simulink model "Appl_VentAdj_CtrlModel"  (R2018b)
settings: configuration reference "CodeConfig_10_ms" (kept outside this file)
undefined symbols (not defined in the file): D_VENT_LVL_1_PRECENT, D_VENT_LVL_2_PRECENT, D_VENT_LVL_3_PRECENT, FALSE, TRUE
libraries: DareLib x72, simulink x1
(part 2 of 4)

== system Appl_VentAdj_CtrlModel/LogicCtrl/LocalAdjustCtrl/LimitDeal/LevelLimitFunction2 ==
  OriginalLevel : Inport
  Error : Inport  Port=2
  OppositeCmd : Inport  Port=3
  CarType : Inport  Port=4
  Vent_CanMessageLostFlag : Inport  Port=5
  Vent_RecoverDefaultFlag : Inport  Port=6
  f : TriggerPort  TriggerType=function-call  VariantControl=(inherit)
      settings: CopyFcn=Stateflow.SLINSF.SimulinkMan.removeBlockPreDeleteFcn  PreDeleteFcn=Stateflow.SLINSF.SimulinkMan.unsafePredeleteFcn
  LevelLimit : Stateflow chart  TreatAsAtomicUnit=on
  Level : Outport
  StopReason : Outport  Port=2
  wires:
  OriginalLevel/1 -> LevelLimit/1(OriginalLevel)
  Error/1 -> LevelLimit/2(Error)
  CarType/1 -> LevelLimit/3(CarType)
  OppositeCmd/1 -> LevelLimit/4(OppositeCmd)
  Vent_CanMessageLostFlag/1 -> LevelLimit/5(Vent_CanMessageLostFlag)
  Vent_RecoverDefaultFlag/1 -> LevelLimit/6(Vent_RecoverDefaultFlag)
  LevelLimit/1(Level) -> Level/1
  LevelLimit/2(StopReason) -> StopReason/1

== system Appl_VentAdj_CtrlModel/LogicCtrl/LocalAdjustCtrl/LimitDeal/MixConflic ==
  MixFlg : Inport  OutDataTypeStr=uint8
  Valid : Inport  Port=2  OutDataTypeStr=uint8
  f : TriggerPort  TriggerType=function-call  VariantControl=(inherit)
      settings: CopyFcn=Stateflow.SLINSF.SimulinkMan.removeBlockPreDeleteFcn  PreDeleteFcn=Stateflow.SLINSF.SimulinkMan.unsafePredeleteFcn
  Constant : Constant  Value=FALSE
  Switch : Switch  Criteria=u2 ~= 0  OutDataTypeStr=uint8
  OutValid : Outport
  wires:
  MixFlg/1 -> Switch/2
  Constant/1 -> Switch/1
  Valid/1 -> Switch/3
  Switch/1 -> OutValid/1

== system Appl_VentAdj_CtrlModel/LogicCtrl/LocalAdjustCtrl/LimitDeal/StopFunction ==
  ComStop : Inport
  Timeout : Inport  Port=2
  f : TriggerPort  TriggerType=function-call  VariantControl=(inherit)
      settings: CopyFcn=Stateflow.SLINSF.SimulinkMan.removeBlockPreDeleteFcn  PreDeleteFcn=Stateflow.SLINSF.SimulinkMan.unsafePredeleteFcn
  StopFunction : Stateflow chart  TreatAsAtomicUnit=on
  StopReason : Outport
  wires:
  Timeout/1 -> StopFunction/1(Timeout)
  ComStop/1 -> StopFunction/2(ComStop)
  StopFunction/1(StopReason) -> StopReason/1

== system Appl_VentAdj_CtrlModel/LogicCtrl/LocalAdjustCtrl/LimitDeal/StopFunction1 ==
  ComStop : Inport
  Timeout : Inport  Port=2
  f : TriggerPort  TriggerType=function-call  VariantControl=(inherit)
      settings: CopyFcn=Stateflow.SLINSF.SimulinkMan.removeBlockPreDeleteFcn  PreDeleteFcn=Stateflow.SLINSF.SimulinkMan.unsafePredeleteFcn
  StopFunction : Stateflow chart  TreatAsAtomicUnit=on
  StopReason : Outport
  wires:
  Timeout/1 -> StopFunction/1(Timeout)
  ComStop/1 -> StopFunction/2(ComStop)
  StopFunction/1(StopReason) -> StopReason/1

== system Appl_VentAdj_CtrlModel/LogicCtrl/LocalAdjustCtrl/LimitDeal/StopFunction2 ==
  ComStop : Inport
  Timeout : Inport  Port=2
  f : TriggerPort  TriggerType=function-call  VariantControl=(inherit)
      settings: CopyFcn=Stateflow.SLINSF.SimulinkMan.removeBlockPreDeleteFcn  PreDeleteFcn=Stateflow.SLINSF.SimulinkMan.unsafePredeleteFcn
  StopFunction : Stateflow chart  TreatAsAtomicUnit=on
  StopReason : Outport
  wires:
  Timeout/1 -> StopFunction/1(Timeout)
  ComStop/1 -> StopFunction/2(ComStop)
  StopFunction/1(StopReason) -> StopReason/1

== system Appl_VentAdj_CtrlModel/LogicCtrl/LocalAdjustCtrl/LimitDeal/TimeoutFunction ==
  TimeoutPrm : Inport
  MaxTime : Inport  Port=2  OutDataTypeStr=uint32
  InLevel : Inport  Port=3
  f : TriggerPort  TriggerType=function-call  VariantControl=(inherit)
      settings: CopyFcn=Stateflow.SLINSF.SimulinkMan.removeBlockPreDeleteFcn  PreDeleteFcn=Stateflow.SLINSF.SimulinkMan.unsafePredeleteFcn
  Timeout : Stateflow chart  TreatAsAtomicUnit=on
  Level : Outport
  TimeoutFlag : Outport  Port=2
  wires:
  TimeoutPrm/1 -> Timeout/1(TimeoutPrm)
  InLevel/1 -> Timeout/2(InLevel)
  Timeout/2(Level) -> Level/1
  Timeout/1(TimeoutFlag) -> TimeoutFlag/1
  MaxTime/1 -> Timeout/3(MaxTime)

== system Appl_VentAdj_CtrlModel/LogicCtrl/LocalAdjustCtrl/LimitDeal/TimeoutFunction1 ==
  TimeoutPrm : Inport
  MaxTime : Inport  Port=2  OutDataTypeStr=uint32
  InLevel : Inport  Port=3
  f : TriggerPort  TriggerType=function-call  VariantControl=(inherit)
      settings: CopyFcn=Stateflow.SLINSF.SimulinkMan.removeBlockPreDeleteFcn  PreDeleteFcn=Stateflow.SLINSF.SimulinkMan.unsafePredeleteFcn
  Timeout : Stateflow chart  TreatAsAtomicUnit=on
  Level : Outport
  TimeoutFlag : Outport  Port=2
  wires:
  TimeoutPrm/1 -> Timeout/1(TimeoutPrm)
  InLevel/1 -> Timeout/2(InLevel)
  Timeout/2(Level) -> Level/1
  Timeout/1(TimeoutFlag) -> TimeoutFlag/1
  MaxTime/1 -> Timeout/3(MaxTime)

== system Appl_VentAdj_CtrlModel/LogicCtrl/LocalAdjustCtrl/LimitDeal/TimeoutFunction2 ==
  TimeoutPrm : Inport
  MaxTime : Inport  Port=2  OutDataTypeStr=uint32
  InLevel : Inport  Port=3
  f : TriggerPort  TriggerType=function-call  VariantControl=(inherit)
      settings: CopyFcn=Stateflow.SLINSF.SimulinkMan.removeBlockPreDeleteFcn  PreDeleteFcn=Stateflow.SLINSF.SimulinkMan.unsafePredeleteFcn
  Timeout : Stateflow chart  TreatAsAtomicUnit=on
  Level : Outport
  TimeoutFlag : Outport  Port=2
  wires:
  TimeoutPrm/1 -> Timeout/1(TimeoutPrm)
  InLevel/1 -> Timeout/2(InLevel)
  Timeout/2(Level) -> Level/1
  Timeout/1(TimeoutFlag) -> TimeoutFlag/1
  MaxTime/1 -> Timeout/3(MaxTime)

== system Appl_VentAdj_CtrlModel/LogicCtrl/LocalAdjustCtrl/OutputDeal/DutyFunction ==
  AimLevel : Inport
  f : TriggerPort  TriggerType=function-call  VariantControl=(inherit)
      settings: CopyFcn=Stateflow.SLINSF.SimulinkMan.removeBlockPreDeleteFcn  PreDeleteFcn=Stateflow.SLINSF.SimulinkMan.unsafePredeleteFcn
  Duty : Stateflow chart  TreatAsAtomicUnit=on
  AimDuty : Outport
  wires:
  AimLevel/1 -> Duty/1(AimLevel)
  Duty/1(AimDuty) -> AimDuty/1

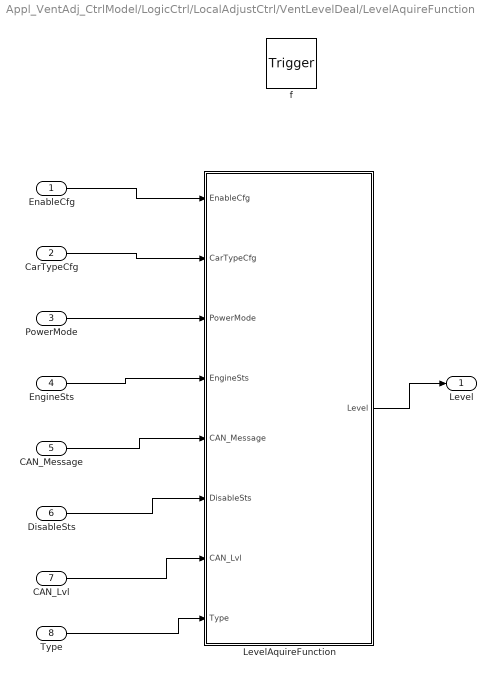
== system Appl_VentAdj_CtrlModel/LogicCtrl/LocalAdjustCtrl/VentLevelDeal/LevelAquireFunction ==
  EnableCfg : Inport
  CarTypeCfg : Inport  Port=2
  PowerMode : Inport  Port=3
  EngineSts : Inport  Port=4
  CAN_Message : Inport  Port=5
  DisableSts : Inport  Port=6
  CAN_Lvl : Inport  Port=7
  Type : Inport  Port=8  OutDataTypeStr=uint8
  f : TriggerPort  TriggerType=function-call  VariantControl=(inherit)
      settings: CopyFcn=Stateflow.SLINSF.SimulinkMan.removeBlockPreDeleteFcn  PreDeleteFcn=Stateflow.SLINSF.SimulinkMan.unsafePredeleteFcn
  LevelAquireFunction : Stateflow chart  TreatAsAtomicUnit=on
  "Level " : Outport
  wires:
  EnableCfg/1 -> LevelAquireFunction/1(EnableCfg)
  DisableSts/1 -> LevelAquireFunction/6(DisableSts)
  CarTypeCfg/1 -> LevelAquireFunction/2(CarTypeCfg)
  CAN_Message/1 -> LevelAquireFunction/5(CAN_Message)
  EngineSts/1 -> LevelAquireFunction/4(EngineSts)
  PowerMode/1 -> LevelAquireFunction/3(PowerMode)
  LevelAquireFunction/1(Level) -> "Level "/1
  CAN_Lvl/1 -> LevelAquireFunction/7(CAN_Lvl)
  Type/1 -> LevelAquireFunction/8(Type)

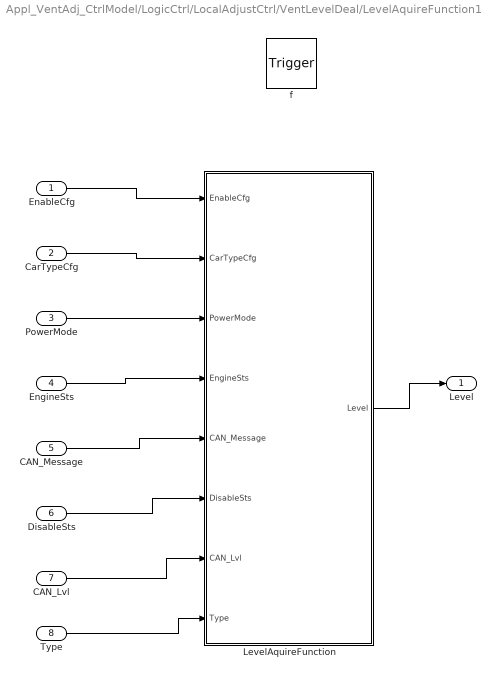
== system Appl_VentAdj_CtrlModel/LogicCtrl/LocalAdjustCtrl/VentLevelDeal/LevelAquireFunction1 ==
  EnableCfg : Inport
  CarTypeCfg : Inport  Port=2
  PowerMode : Inport  Port=3
  EngineSts : Inport  Port=4
  CAN_Message : Inport  Port=5
  DisableSts : Inport  Port=6
  CAN_Lvl : Inport  Port=7
  Type : Inport  Port=8  OutDataTypeStr=uint8
  f : TriggerPort  TriggerType=function-call  VariantControl=(inherit)
      settings: CopyFcn=Stateflow.SLINSF.SimulinkMan.removeBlockPreDeleteFcn  PreDeleteFcn=Stateflow.SLINSF.SimulinkMan.unsafePredeleteFcn
  LevelAquireFunction : Stateflow chart  TreatAsAtomicUnit=on
  "Level " : Outport
  wires:
  EnableCfg/1 -> LevelAquireFunction/1(EnableCfg)
  DisableSts/1 -> LevelAquireFunction/6(DisableSts)
  CarTypeCfg/1 -> LevelAquireFunction/2(CarTypeCfg)
  CAN_Message/1 -> LevelAquireFunction/5(CAN_Message)
  EngineSts/1 -> LevelAquireFunction/4(EngineSts)
  PowerMode/1 -> LevelAquireFunction/3(PowerMode)
  LevelAquireFunction/1(Level) -> "Level "/1
  CAN_Lvl/1 -> LevelAquireFunction/7(CAN_Lvl)
  Type/1 -> LevelAquireFunction/8(Type)

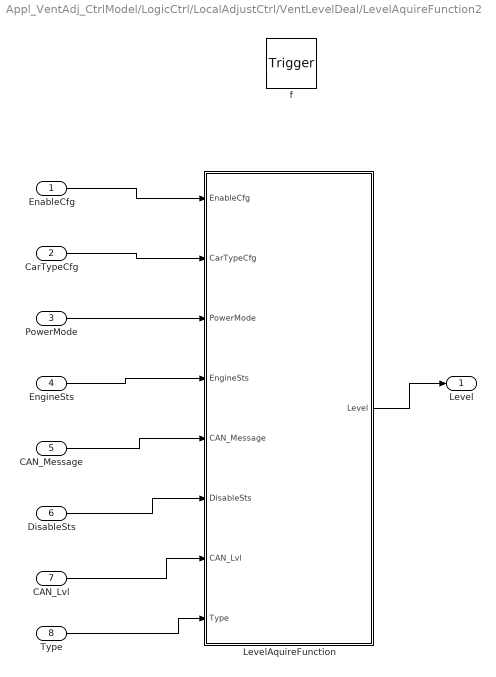
== system Appl_VentAdj_CtrlModel/LogicCtrl/LocalAdjustCtrl/VentLevelDeal/LevelAquireFunction2 ==
  EnableCfg : Inport
  CarTypeCfg : Inport  Port=2
  PowerMode : Inport  Port=3
  EngineSts : Inport  Port=4
  CAN_Message : Inport  Port=5
  DisableSts : Inport  Port=6
  CAN_Lvl : Inport  Port=7
  Type : Inport  Port=8  OutDataTypeStr=uint8
  f : TriggerPort  TriggerType=function-call  VariantControl=(inherit)
      settings: CopyFcn=Stateflow.SLINSF.SimulinkMan.removeBlockPreDeleteFcn  PreDeleteFcn=Stateflow.SLINSF.SimulinkMan.unsafePredeleteFcn
  LevelAquireFunction : Stateflow chart  TreatAsAtomicUnit=on
  "Level " : Outport
  wires:
  EnableCfg/1 -> LevelAquireFunction/1(EnableCfg)
  DisableSts/1 -> LevelAquireFunction/6(DisableSts)
  CarTypeCfg/1 -> LevelAquireFunction/2(CarTypeCfg)
  CAN_Message/1 -> LevelAquireFunction/5(CAN_Message)
  EngineSts/1 -> LevelAquireFunction/4(EngineSts)
  PowerMode/1 -> LevelAquireFunction/3(PowerMode)
  LevelAquireFunction/1(Level) -> "Level "/1
  CAN_Lvl/1 -> LevelAquireFunction/7(CAN_Lvl)
  Type/1 -> LevelAquireFunction/8(Type)

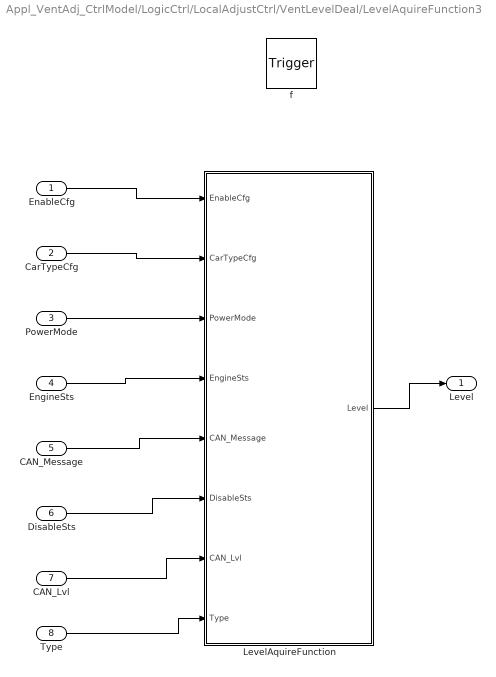
== system Appl_VentAdj_CtrlModel/LogicCtrl/LocalAdjustCtrl/VentLevelDeal/LevelAquireFunction3 ==
  EnableCfg : Inport
  CarTypeCfg : Inport  Port=2
  PowerMode : Inport  Port=3
  EngineSts : Inport  Port=4
  CAN_Message : Inport  Port=5
  DisableSts : Inport  Port=6
  CAN_Lvl : Inport  Port=7
  Type : Inport  Port=8  OutDataTypeStr=uint8
  f : TriggerPort  TriggerType=function-call  VariantControl=(inherit)
      settings: CopyFcn=Stateflow.SLINSF.SimulinkMan.removeBlockPreDeleteFcn  PreDeleteFcn=Stateflow.SLINSF.SimulinkMan.unsafePredeleteFcn
  LevelAquireFunction : Stateflow chart  TreatAsAtomicUnit=on
  "Level " : Outport
  wires:
  EnableCfg/1 -> LevelAquireFunction/1(EnableCfg)
  DisableSts/1 -> LevelAquireFunction/6(DisableSts)
  CarTypeCfg/1 -> LevelAquireFunction/2(CarTypeCfg)
  CAN_Message/1 -> LevelAquireFunction/5(CAN_Message)
  EngineSts/1 -> LevelAquireFunction/4(EngineSts)
  PowerMode/1 -> LevelAquireFunction/3(PowerMode)
  LevelAquireFunction/1(Level) -> "Level "/1
  CAN_Lvl/1 -> LevelAquireFunction/7(CAN_Lvl)
  Type/1 -> LevelAquireFunction/8(Type)

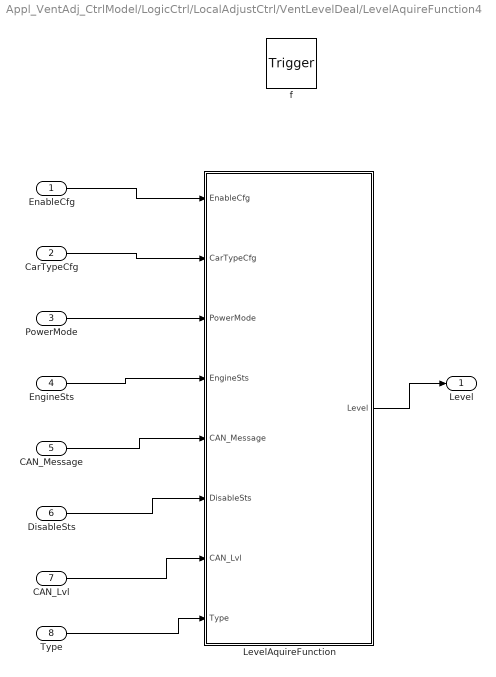
== system Appl_VentAdj_CtrlModel/LogicCtrl/LocalAdjustCtrl/VentLevelDeal/LevelAquireFunction4 ==
  EnableCfg : Inport
  CarTypeCfg : Inport  Port=2
  PowerMode : Inport  Port=3
  EngineSts : Inport  Port=4
  CAN_Message : Inport  Port=5
  DisableSts : Inport  Port=6
  CAN_Lvl : Inport  Port=7
  Type : Inport  Port=8  OutDataTypeStr=uint8
  f : TriggerPort  TriggerType=function-call  VariantControl=(inherit)
      settings: CopyFcn=Stateflow.SLINSF.SimulinkMan.removeBlockPreDeleteFcn  PreDeleteFcn=Stateflow.SLINSF.SimulinkMan.unsafePredeleteFcn
  LevelAquireFunction : Stateflow chart  TreatAsAtomicUnit=on
  "Level " : Outport
  wires:
  EnableCfg/1 -> LevelAquireFunction/1(EnableCfg)
  DisableSts/1 -> LevelAquireFunction/6(DisableSts)
  CarTypeCfg/1 -> LevelAquireFunction/2(CarTypeCfg)
  CAN_Message/1 -> LevelAquireFunction/5(CAN_Message)
  EngineSts/1 -> LevelAquireFunction/4(EngineSts)
  PowerMode/1 -> LevelAquireFunction/3(PowerMode)
  LevelAquireFunction/1(Level) -> "Level "/1
  CAN_Lvl/1 -> LevelAquireFunction/7(CAN_Lvl)
  Type/1 -> LevelAquireFunction/8(Type)

== system Appl_VentAdj_CtrlModel/LogicCtrl/LocalAdjustCtrl/VentLevelDeal/LevelAquireFunction5 ==
  EnableCfg : Inport
  CarTypeCfg : Inport  Port=2
  PowerMode : Inport  Port=3
  EngineSts : Inport  Port=4
  CAN_Message : Inport  Port=5
  DisableSts : Inport  Port=6
  CAN_Lvl : Inport  Port=7
  Type : Inport  Port=8  OutDataTypeStr=uint8
  f : TriggerPort  TriggerType=function-call  VariantControl=(inherit)
      settings: CopyFcn=Stateflow.SLINSF.SimulinkMan.removeBlockPreDeleteFcn  PreDeleteFcn=Stateflow.SLINSF.SimulinkMan.unsafePredeleteFcn
  LevelAquireFunction : Stateflow chart  TreatAsAtomicUnit=on
  "Level " : Outport
  wires:
  EnableCfg/1 -> LevelAquireFunction/1(EnableCfg)
  DisableSts/1 -> LevelAquireFunction/6(DisableSts)
  CarTypeCfg/1 -> LevelAquireFunction/2(CarTypeCfg)
  CAN_Message/1 -> LevelAquireFunction/5(CAN_Message)
  EngineSts/1 -> LevelAquireFunction/4(EngineSts)
  PowerMode/1 -> LevelAquireFunction/3(PowerMode)
  LevelAquireFunction/1(Level) -> "Level "/1
  CAN_Lvl/1 -> LevelAquireFunction/7(CAN_Lvl)
  Type/1 -> LevelAquireFunction/8(Type)

== system Appl_VentAdj_CtrlModel/LogicCtrl/LocalAdjustCtrl/VentLevelDeal/VentRunTypeFunction ==
  InLevel : Inport
  PreLevel : Inport  Port=2
  InType : Inport  Port=3
  f : TriggerPort  TriggerType=function-call  VariantControl=(inherit)
      settings: CopyFcn=Stateflow.SLINSF.SimulinkMan.removeBlockPreDeleteFcn  PreDeleteFcn=Stateflow.SLINSF.SimulinkMan.unsafePredeleteFcn
  VentRunType : Stateflow chart  TreatAsAtomicUnit=on
  RunType : Outport
  OutLevel : Outport  Port=2
  wires:
  InLevel/1 -> VentRunType/1(InLevel)
  PreLevel/1 -> VentRunType/2(PreLevel)
  InType/1 -> VentRunType/3(InType)
  VentRunType/1(RunType) -> RunType/1
  VentRunType/2(OutLevel) -> OutLevel/1

== system Appl_VentAdj_CtrlModel/UpDataInputInfo/InputSignalProcess/CommonPreconditionDeal ==
  EngineRunningFlag : Inport
  VehicleRunFlag : Inport  Port=2
  VentAdj_VoltMode : Inport  Port=3
  Deal : Stateflow chart  TreatAsAtomicUnit=on
  "ComPCSatisfiedFlag " : Outport
  wires:
  EngineRunningFlag/1 -> Deal/1(EngineRunningFlag)
  VehicleRunFlag/1 -> Deal/2(VehicleRunFlag)
  Deal/1(ComPCSatisfiedFlag) -> "ComPCSatisfiedFlag "/1
  VentAdj_VoltMode/1 -> Deal/3(VentAdj_VoltMode)

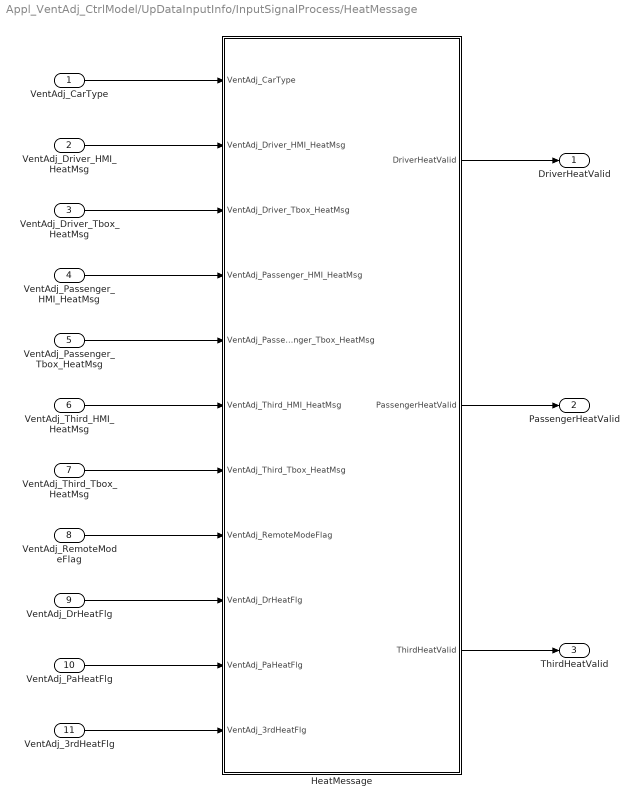
== system Appl_VentAdj_CtrlModel/UpDataInputInfo/InputSignalProcess/HeatMessage ==
  VentAdj_CarType : Inport
  VentAdj_Driver_HMI_HeatMsg : Inport  Port=2
  VentAdj_Driver_Tbox_HeatMsg : Inport  Port=3
  VentAdj_Passenger_HMI_HeatMsg : Inport  Port=4
  VentAdj_Passenger_Tbox_HeatMsg : Inport  Port=5
  VentAdj_Third_HMI_HeatMsg : Inport  Port=6
  VentAdj_Third_Tbox_HeatMsg : Inport  Port=7
  VentAdj_RemoteModeFlag : Inport  Port=8
  VentAdj_DrHeatFlg : Inport  Port=9
  VentAdj_PaHeatFlg : Inport  Port=10
  VentAdj_3rdHeatFlg : Inport  Port=11
  HeatMessage : Stateflow chart  TreatAsAtomicUnit=on
  DriverHeatValid : Outport
  PassengerHeatValid : Outport  Port=2
  ThirdHeatValid : Outport  Port=3
  wires:
  VentAdj_Driver_HMI_HeatMsg/1 -> HeatMessage/2(VentAdj_Driver_HMI_HeatMsg)
  VentAdj_CarType/1 -> HeatMessage/1(VentAdj_CarType)
  VentAdj_Driver_Tbox_HeatMsg/1 -> HeatMessage/3(VentAdj_Driver_Tbox_HeatMsg)
  VentAdj_Passenger_HMI_HeatMsg/1 -> HeatMessage/4(VentAdj_Passenger_HMI_HeatMsg)
  VentAdj_Passenger_Tbox_HeatMsg/1 -> HeatMessage/5(VentAdj_Passenger_Tbox_HeatMsg)
  VentAdj_RemoteModeFlag/1 -> HeatMessage/8(VentAdj_RemoteModeFlag)
  VentAdj_Third_HMI_HeatMsg/1 -> HeatMessage/6(VentAdj_Third_HMI_HeatMsg)
  VentAdj_Third_Tbox_HeatMsg/1 -> HeatMessage/7(VentAdj_Third_Tbox_HeatMsg)
  HeatMessage/1(DriverHeatValid) -> DriverHeatValid/1
  HeatMessage/2(PassengerHeatValid) -> PassengerHeatValid/1
  HeatMessage/3(ThirdHeatValid) -> ThirdHeatValid/1
  VentAdj_DrHeatFlg/1 -> HeatMessage/9(VentAdj_DrHeatFlg)
  VentAdj_PaHeatFlg/1 -> HeatMessage/10(VentAdj_PaHeatFlg)
  VentAdj_3rdHeatFlg/1 -> HeatMessage/11(VentAdj_3rdHeatFlg)

== system Appl_VentAdj_CtrlModel/UpDataInputInfo/InputSignalProcess/MaxTime ==
  VentAdj_CarType : Inport
  Constant : Constant  Value=60  OutDataTypeStr=uint32
  Constant1 : Constant  Value=1000  OutDataTypeStr=uint32
  Constant5 : Constant  Value=[0 0]  OutDataTypeStr=uint32
  Product : Product  Inputs=3  OutDataTypeStr=uint32
  Selector5 : Selector  IndexMode=Zero-based  InputPortWidth=2  IndexOptions=Index vector (port)  Indices=[1 3]  OutputSizes=1
  TimeChangeToCycle5 : DareLib/Dare/TimeChangeToCycle  Description=时间转成执行周期  Commented=on  Sec=60  Msec=1000  Cycle=CAL_HeatAdjCycle_10ms
      settings: AttributesFormatString=%<Description>  SourceProductName=Dare Library
  VentRunMaxTime : Outport
  wires:
  VentAdj_CarType/1 -> Selector5/2
  Constant5/1 -> Selector5/1
  Selector5/1 -> Product/2
  Constant/1 -> Product/1
  Constant1/1 -> Product/3
  Product/1 -> VentRunMaxTime/1

== system Appl_VentAdj_CtrlModel/UpDataInputInfo/InputSignalProcess/Subsystem ==
  VentAdj_DriverEnableConfig : Inport
  VentAdj_PassengerEnableConfig : Inport  Port=2
  VentAdj_ThirdEnableConfig : Inport  Port=3
  VentAdj_DrVentFlg : Inport  Port=4
  VentAdj_PaVentFlg : Inport  Port=5
  Bus Creator : BusCreator  Inputs=3
  Logical Operator : Logic  AllPortsSameDT=off  OutDataTypeStr=boolean
  Logical Operator1 : Logic  AllPortsSameDT=off  OutDataTypeStr=boolean
  VentEnable : Outport
  wires:
  Bus Creator/1 -> VentEnable/1
  VentAdj_DriverEnableConfig/1 -> Logical Operator1/1
  Logical Operator1/1 -> Bus Creator/1  "DrvVentFlg"
  VentAdj_PaVentFlg/1 -> Logical Operator/2
  VentAdj_PassengerEnableConfig/1 -> Logical Operator/1
  Logical Operator/1 -> Bus Creator/2  "PaVentFlg"
  VentAdj_ThirdEnableConfig/1 -> Bus Creator/3  "ThirdVentFlg"
  VentAdj_DrVentFlg/1 -> Logical Operator1/2

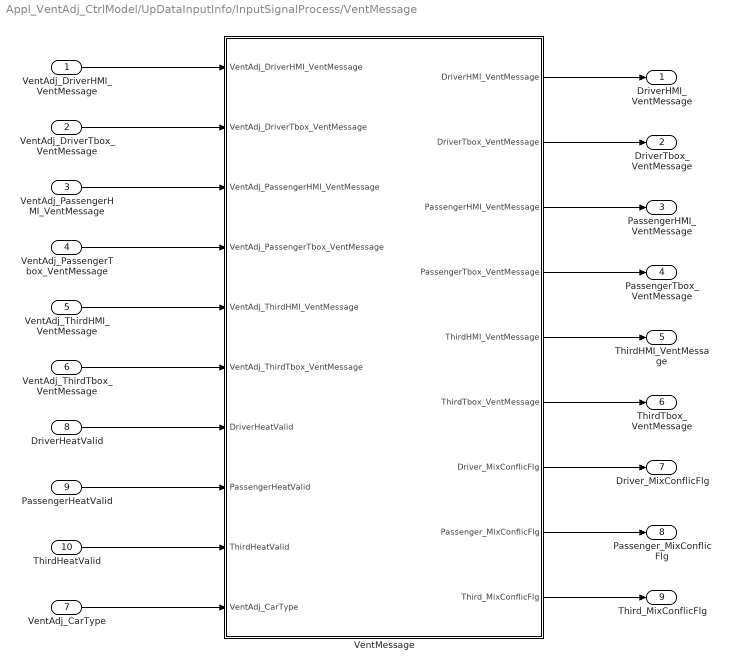
== system Appl_VentAdj_CtrlModel/UpDataInputInfo/InputSignalProcess/VentMessage ==
  VentAdj_DriverHMI_VentMessage : Inport
  VentAdj_DriverTbox_VentMessage : Inport  Port=2
  VentAdj_PassengerHMI_VentMessage : Inport  Port=3
  VentAdj_PassengerTbox_VentMessage : Inport  Port=4
  VentAdj_ThirdHMI_VentMessage : Inport  Port=5
  VentAdj_ThirdTbox_VentMessage : Inport  Port=6
  VentAdj_CarType : Inport  Port=7
  DriverHeatValid : Inport  Port=8
  PassengerHeatValid : Inport  Port=9
  ThirdHeatValid : Inport  Port=10
  VentMessage : Stateflow chart  TreatAsAtomicUnit=on
  DriverHMI_VentMessage : Outport
  DriverTbox_VentMessage : Outport  Port=2
  PassengerHMI_VentMessage : Outport  Port=3
  PassengerTbox_VentMessage : Outport  Port=4
  ThirdHMI_VentMessage : Outport  Port=5
  ThirdTbox_VentMessage : Outport  Port=6
  Driver_MixConflicFlg : Outport  Port=7
  Passenger_MixConflicFlg : Outport  Port=8
  Third_MixConflicFlg : Outport  Port=9
  wires:
  VentMessage/3(PassengerHMI_VentMessage) -> PassengerHMI_VentMessage/1
  VentMessage/2(DriverTbox_VentMessage) -> DriverTbox_VentMessage/1
  VentMessage/1(DriverHMI_VentMessage) -> DriverHMI_VentMessage/1
  DriverHeatValid/1 -> VentMessage/7(DriverHeatValid)
  VentAdj_ThirdTbox_VentMessage/1 -> VentMessage/6(VentAdj_ThirdTbox_VentMessage)
  PassengerHeatValid/1 -> VentMessage/8(PassengerHeatValid)
  VentAdj_ThirdHMI_VentMessage/1 -> VentMessage/5(VentAdj_ThirdHMI_VentMessage)
  VentAdj_PassengerTbox_VentMessage/1 -> VentMessage/4(VentAdj_PassengerTbox_VentMessage)
  VentAdj_PassengerHMI_VentMessage/1 -> VentMessage/3(VentAdj_PassengerHMI_VentMessage)
  VentAdj_DriverHMI_VentMessage/1 -> VentMessage/1(VentAdj_DriverHMI_VentMessage)
  VentAdj_DriverTbox_VentMessage/1 -> VentMessage/2(VentAdj_DriverTbox_VentMessage)
  ThirdHeatValid/1 -> VentMessage/9(ThirdHeatValid)
  VentMessage/6(ThirdTbox_VentMessage) -> ThirdTbox_VentMessage/1
  VentMessage/5(ThirdHMI_VentMessage) -> ThirdHMI_VentMessage/1
  VentMessage/4(PassengerTbox_VentMessage) -> PassengerTbox_VentMessage/1
  VentAdj_CarType/1 -> VentMessage/10(VentAdj_CarType)
  VentMessage/7(Driver_MixConflicFlg) -> Driver_MixConflicFlg/1
  VentMessage/8(Passenger_MixConflicFlg) -> Passenger_MixConflicFlg/1
  VentMessage/9(Third_MixConflicFlg) -> Third_MixConflicFlg/1

== system Appl_VentAdj_CtrlModel/LogicCtrl/LocalAdjustCtrl/LimitDeal/TimeoutFunction/Timeout/D_HAL_GET_CUR_MS_TS ==
  f : TriggerPort  TriggerType=function-call  VariantControl=(inherit)
      settings: CopyFcn=Stateflow.SLINSF.SimulinkMan.removeBlockPreDeleteFcn  PreDeleteFcn=Stateflow.SLINSF.SimulinkMan.unsafePredeleteFcn
  DrAdj_LenAdjSize : DareLib/Dare/getAPI_type  g_funcname=D_HAL_GET_CUR_MS_TS  g_param=""  g_type=uint32  g_size=-1
      settings: SourceProductName=Dare Library
  Ts : Outport
  wires:
  DrAdj_LenAdjSize/1 -> Ts/1  "D_HAL_GET_CUR_MS_TS"

== system Appl_VentAdj_CtrlModel/LogicCtrl/LocalAdjustCtrl/LimitDeal/TimeoutFunction/Timeout/TimeDiffTs ==
  lastTs : Inport
  Ts : Inport  Port=2
  f : TriggerPort  TriggerType=function-call  VariantControl=(inherit)
      settings: CopyFcn=Stateflow.SLINSF.SimulinkMan.removeBlockPreDeleteFcn  PreDeleteFcn=Stateflow.SLINSF.SimulinkMan.unsafePredeleteFcn
  Chart : Stateflow chart  TreatAsAtomicUnit=on
  OutTs : Outport
  wires:
  lastTs/1 -> Chart/1(lastTs)
  Ts/1 -> Chart/2(Ts)
  Chart/1(OutTs) -> OutTs/1

== system Appl_VentAdj_CtrlModel/LogicCtrl/LocalAdjustCtrl/LimitDeal/TimeoutFunction1/Timeout/D_HAL_GET_CUR_MS_TS ==
  f : TriggerPort  TriggerType=function-call  VariantControl=(inherit)
      settings: CopyFcn=Stateflow.SLINSF.SimulinkMan.removeBlockPreDeleteFcn  PreDeleteFcn=Stateflow.SLINSF.SimulinkMan.unsafePredeleteFcn
  DrAdj_LenAdjSize : DareLib/Dare/getAPI_type  g_funcname=D_HAL_GET_CUR_MS_TS  g_param=""  g_type=uint32  g_size=-1
      settings: SourceProductName=Dare Library
  Ts : Outport
  wires:
  DrAdj_LenAdjSize/1 -> Ts/1  "D_HAL_GET_CUR_MS_TS"

== system Appl_VentAdj_CtrlModel/LogicCtrl/LocalAdjustCtrl/LimitDeal/TimeoutFunction1/Timeout/TimeDiffTs ==
  lastTs : Inport
  Ts : Inport  Port=2
  f : TriggerPort  TriggerType=function-call  VariantControl=(inherit)
      settings: CopyFcn=Stateflow.SLINSF.SimulinkMan.removeBlockPreDeleteFcn  PreDeleteFcn=Stateflow.SLINSF.SimulinkMan.unsafePredeleteFcn
  Chart : Stateflow chart  TreatAsAtomicUnit=on
  OutTs : Outport
  wires:
  lastTs/1 -> Chart/1(lastTs)
  Ts/1 -> Chart/2(Ts)
  Chart/1(OutTs) -> OutTs/1

== system Appl_VentAdj_CtrlModel/LogicCtrl/LocalAdjustCtrl/LimitDeal/TimeoutFunction2/Timeout/D_HAL_GET_CUR_MS_TS ==
  f : TriggerPort  TriggerType=function-call  VariantControl=(inherit)
      settings: CopyFcn=Stateflow.SLINSF.SimulinkMan.removeBlockPreDeleteFcn  PreDeleteFcn=Stateflow.SLINSF.SimulinkMan.unsafePredeleteFcn
  DrAdj_LenAdjSize : DareLib/Dare/getAPI_type  g_funcname=D_HAL_GET_CUR_MS_TS  g_param=""  g_type=uint32  g_size=-1
      settings: SourceProductName=Dare Library
  Ts : Outport
  wires:
  DrAdj_LenAdjSize/1 -> Ts/1  "D_HAL_GET_CUR_MS_TS"

== system Appl_VentAdj_CtrlModel/LogicCtrl/LocalAdjustCtrl/LimitDeal/TimeoutFunction2/Timeout/TimeDiffTs ==
  lastTs : Inport
  Ts : Inport  Port=2
  f : TriggerPort  TriggerType=function-call  VariantControl=(inherit)
      settings: CopyFcn=Stateflow.SLINSF.SimulinkMan.removeBlockPreDeleteFcn  PreDeleteFcn=Stateflow.SLINSF.SimulinkMan.unsafePredeleteFcn
  Chart : Stateflow chart  TreatAsAtomicUnit=on
  OutTs : Outport
  wires:
  lastTs/1 -> Chart/1(lastTs)
  Ts/1 -> Chart/2(Ts)
  Chart/1(OutTs) -> OutTs/1

== system Appl_VentAdj_CtrlModel/UpDataInputInfo/InputSignalProcess/HeatMessage/HeatMessage/OppositeMessageDeal ==
  CarTypeCfg : Inport
  RemoteModeFlag : Inport  Port=2
  HMI_Message : Inport  Port=3
  Tbox_Message : Inport  Port=4
  HeatCfg : Inport  Port=5
  f : TriggerPort  TriggerType=function-call  VariantControl=(inherit)
      settings: CopyFcn=Stateflow.SLINSF.SimulinkMan.removeBlockPreDeleteFcn  PreDeleteFcn=Stateflow.SLINSF.SimulinkMan.unsafePredeleteFcn
  OppositeMessageDeal : Stateflow chart  TreatAsAtomicUnit=on
  "VenSts " : Outport
  wires:
  OppositeMessageDeal/1(VenSts) -> "VenSts "/1
  Tbox_Message/1 -> OppositeMessageDeal/4(Tbox_Message)
  CarTypeCfg/1 -> OppositeMessageDeal/1(CarTypeCfg)
  HMI_Message/1 -> OppositeMessageDeal/3(HMI_Message)
  RemoteModeFlag/1 -> OppositeMessageDeal/2(RemoteModeFlag)
  HeatCfg/1 -> OppositeMessageDeal/5(HeatCfg)

== system Appl_VentAdj_CtrlModel/UpDataInputInfo/InputSignalProcess/HeatMessage/HeatMessage/OppositeMessageDeal1 ==
  CarTypeCfg : Inport
  RemoteModeFlag : Inport  Port=2
  HMI_Message : Inport  Port=3
  Tbox_Message : Inport  Port=4
  HeatCfg : Inport  Port=5
  f : TriggerPort  TriggerType=function-call  VariantControl=(inherit)
      settings: CopyFcn=Stateflow.SLINSF.SimulinkMan.removeBlockPreDeleteFcn  PreDeleteFcn=Stateflow.SLINSF.SimulinkMan.unsafePredeleteFcn
  OppositeMessageDeal : Stateflow chart  TreatAsAtomicUnit=on
  "VenSts " : Outport
  wires:
  OppositeMessageDeal/1(VenSts) -> "VenSts "/1
  Tbox_Message/1 -> OppositeMessageDeal/4(Tbox_Message)
  CarTypeCfg/1 -> OppositeMessageDeal/1(CarTypeCfg)
  HMI_Message/1 -> OppositeMessageDeal/3(HMI_Message)
  RemoteModeFlag/1 -> OppositeMessageDeal/2(RemoteModeFlag)
  HeatCfg/1 -> OppositeMessageDeal/5(HeatCfg)

== system Appl_VentAdj_CtrlModel/UpDataInputInfo/InputSignalProcess/HeatMessage/HeatMessage/OppositeMessageDeal2 ==
  CarTypeCfg : Inport
  RemoteModeFlag : Inport  Port=2
  HMI_Message : Inport  Port=3
  Tbox_Message : Inport  Port=4
  HeatCfg : Inport  Port=5
  f : TriggerPort  TriggerType=function-call  VariantControl=(inherit)
      settings: CopyFcn=Stateflow.SLINSF.SimulinkMan.removeBlockPreDeleteFcn  PreDeleteFcn=Stateflow.SLINSF.SimulinkMan.unsafePredeleteFcn
  OppositeMessageDeal : Stateflow chart  TreatAsAtomicUnit=on
  "VenSts " : Outport
  wires:
  OppositeMessageDeal/1(VenSts) -> "VenSts "/1
  Tbox_Message/1 -> OppositeMessageDeal/4(Tbox_Message)
  CarTypeCfg/1 -> OppositeMessageDeal/1(CarTypeCfg)
  HMI_Message/1 -> OppositeMessageDeal/3(HMI_Message)
  RemoteModeFlag/1 -> OppositeMessageDeal/2(RemoteModeFlag)
  HeatCfg/1 -> OppositeMessageDeal/5(HeatCfg)

== system Appl_VentAdj_CtrlModel/UpDataInputInfo/InputSignalProcess/VentMessage/VentMessage/MsgConflictFunction ==
  CarTypeCfg : Inport
  HMI_Message : Inport  Port=2  OutDataTypeStr=uint8
  Tbox_Message : Inport  Port=3  OutDataTypeStr=uint8
  VentValidFlag : Inport  Port=4
  f : TriggerPort  TriggerType=function-call  VariantControl=(inherit)
      settings: CopyFcn=Stateflow.SLINSF.SimulinkMan.removeBlockPreDeleteFcn  PreDeleteFcn=Stateflow.SLINSF.SimulinkMan.unsafePredeleteFcn
  Function : Stateflow chart  TreatAsAtomicUnit=on
  OutMsgHMI : Outport
  OutMsgTbox : Outport  Port=2
  MixConflictFlg : Outport  Port=3
  wires:
  Function/1(OutMsgHMI) -> OutMsgHMI/1
  VentValidFlag/1 -> Function/4(VentValidFlag)
  CarTypeCfg/1 -> Function/1(CarTypeCfg)
  HMI_Message/1 -> Function/2(HMI_Message)
  Tbox_Message/1 -> Function/3(Tbox_Message)
  Function/2(OutMsgTbox) -> OutMsgTbox/1
  Function/3(MixConflictFlg) -> MixConflictFlg/1

== system Appl_VentAdj_CtrlModel/UpDataInputInfo/InputSignalProcess/VentMessage/VentMessage/MsgConflictFunction1 ==
  CarTypeCfg : Inport
  HMI_Message : Inport  Port=2  OutDataTypeStr=uint8
  Tbox_Message : Inport  Port=3  OutDataTypeStr=uint8
  VentValidFlag : Inport  Port=4
  f : TriggerPort  TriggerType=function-call  VariantControl=(inherit)
      settings: CopyFcn=Stateflow.SLINSF.SimulinkMan.removeBlockPreDeleteFcn  PreDeleteFcn=Stateflow.SLINSF.SimulinkMan.unsafePredeleteFcn
  Function : Stateflow chart  TreatAsAtomicUnit=on
  OutMsgHMI : Outport
  OutMsgTbox : Outport  Port=2
  MixConflictFlg : Outport  Port=3
  wires:
  Function/1(OutMsgHMI) -> OutMsgHMI/1
  VentValidFlag/1 -> Function/4(VentValidFlag)
  CarTypeCfg/1 -> Function/1(CarTypeCfg)
  HMI_Message/1 -> Function/2(HMI_Message)
  Tbox_Message/1 -> Function/3(Tbox_Message)
  Function/2(OutMsgTbox) -> OutMsgTbox/1
  Function/3(MixConflictFlg) -> MixConflictFlg/1

== system Appl_VentAdj_CtrlModel/UpDataInputInfo/InputSignalProcess/VentMessage/VentMessage/MsgConflictFunction2 ==
  CarTypeCfg : Inport
  HMI_Message : Inport  Port=2  OutDataTypeStr=uint8
  Tbox_Message : Inport  Port=3  OutDataTypeStr=uint8
  VentValidFlag : Inport  Port=4
  f : TriggerPort  TriggerType=function-call  VariantControl=(inherit)
      settings: CopyFcn=Stateflow.SLINSF.SimulinkMan.removeBlockPreDeleteFcn  PreDeleteFcn=Stateflow.SLINSF.SimulinkMan.unsafePredeleteFcn
  Function : Stateflow chart  TreatAsAtomicUnit=on
  OutMsgHMI : Outport
  OutMsgTbox : Outport  Port=2
  MixConflictFlg : Outport  Port=3
  wires:
  Function/1(OutMsgHMI) -> OutMsgHMI/1
  VentValidFlag/1 -> Function/4(VentValidFlag)
  CarTypeCfg/1 -> Function/1(CarTypeCfg)
  HMI_Message/1 -> Function/2(HMI_Message)
  Tbox_Message/1 -> Function/3(Tbox_Message)
  Function/2(OutMsgTbox) -> OutMsgTbox/1
  Function/3(MixConflictFlg) -> MixConflictFlg/1

== stateflow chart Appl_VentAdj_CtrlModel/LogicCtrl/LocalAdjustCtrl/VentLevelDeal/LevelAquireFunction1/LevelAquireFunction ==
  state LevelAquire
    (default) -> (junction 92)
    LevelAquire -> (junction 92)
    (junction 92) -> (junction 95) [order 1] : /*加热功能禁能
        | || OFF 电
        | || 发动机不在运行中*/
        | [enVentStopReason.EN_VENT_STOP_R_NONE != DisableSts ...
        | || FALSE == EnableCfg ...
        | || enPowerModeSts.EN_OFF == PowerMode ...
        | || TRUE != EngineSts]
    (junction 92) -> (junction 94) [order 2] : {StopFlag = FALSE;}
    (junction 95) -> (junction 93) : {Level = enVentLvlSts.EN_VENT_LVL_OFF;
        | StopFlag = TRUE;}
    (junction 93) -> (junction 94)
    (junction 94) -> (junction 101)
    (junction 101) -> (junction 21) [order 1] : [StopFlag == FALSE]
    (junction 21) -> (junction 23) [order 1] : [enProjectType.EN_PROJECT_P20 == CarTypeCfg]
    (junction 101) -> (junction 104) [order 2] : {Level = enVentLvlSts.EN_VENT_LVL_OFF;}
    (junction 21) -> (junction 48) [order 2]
    (junction 23) -> (junction 82)
    (junction 82) -> (junction 84) [order 1] : /* 一键开启 且为Hmi控制 */
        | [5 == CAN_Message && Type == 0]
    (junction 82) -> (junction 25) [order 2]
    (junction 84) -> (junction 86) : {Level = CAN_Lvl + 1;}
    (junction 25) -> (junction 27) [order 1] : [4 == CAN_Message]
    (junction 25) -> (junction 29) [order 2] : {TempMsg = CAN_Message + 7;}
    (junction 27) -> (junction 57) : {Level = enVentLvlSts.EN_VENT_LVL_OFF;}
    (junction 48) -> (junction 50) [order 1] : [1 != CAN_Message]
    (junction 48) -> (junction 55) [order 2] : {Level = enVentLvlSts.EN_VENT_LVL_OFF;}
    (junction 50) -> (junction 52) : {TempMsg = CAN_Message;}
    (junction 52) -> (junction 29)
    (junction 29) -> (junction 32) [order 1] : [7 < TempMsg && 11 > TempMsg]
    (junction 29) -> (junction 36) [order 2] : {Level = 0xFF;}
    (junction 32) -> (junction 34)
    (junction 34) -> (junction 38) [order 1] : [8 == TempMsg]
    (junction 34) -> (junction 40) [order 2]
    (junction 38) -> (junction 59) : {Level = enVentLvlSts.EN_VENT_LVL_1;}
    (junction 40) -> (junction 42) [order 1] : [9 == TempMsg]
    (junction 40) -> (junction 46) [order 2] : {Level = enVentLvlSts.EN_VENT_LVL_3;}
    (junction 42) -> (junction 44) : {Level = enVentLvlSts.EN_VENT_LVL_2;}
    (junction 55) -> (junction 104)
    (junction 36) -> (junction 55)
    (junction 46) -> (junction 36)
    (junction 44) -> (junction 46)
    (junction 59) -> (junction 44)
    (junction 57) -> (junction 59)
    (junction 86) -> (junction 57)
    (junction 104) -> (junction 75)
  data: EnableCfg input uint8; CarTypeCfg input Enum: enProjectType; PowerMode input Enum: enPowerModeSts; EngineSts input uint8; CAN_Message input uint8; DisableSts input Enum: enVentStopReason; Level output uint8; TempMsg local uint8; TRUE parameter; FALSE parameter; CAN_Lvl input uint8; Type input; StopFlag local boolean

== stateflow chart Appl_VentAdj_CtrlModel/LogicCtrl/LocalAdjustCtrl/LimitDeal ==
  state OutValid = MixConflic(MixFlg,Valid) [function]
  state MixConflic1 [parallel]
    en,du:
    [LocalDriverHeatValid] = MixConflic(Driver_MixConflicFlg, DriverHeatValid);
    [LocalPassengerHeatValid] = MixConflic(Passenger_MixConflicFlg, PassengerHeatValid);
    [LocalThirdHeatValid] = MixConflic(Third_MixConflicFlg, ThirdHeatValid);
    settings: executionOrder=1
  state [Level,StopReason] = LevelLimitFunction(OriginalLevel,Error,OppositeCmd,CarType,Vent_CanMessageLostFlag,Vent_RecoverDefaultFlag) [function]
  state ForbidLimitDeal [parallel]
    en,du:
    [ComDrVentLevel,ComDrStopReason] = LevelLimitFunction(OriginalDrVentLevel,VentAdj_DriverCmdFaultSts, LocalDriverHeatValid,VentAdj_CarType,VentAdj_HeatMsgLostFlag,VentAdj_RecoverDefaultFlag);
    [ComPaVentLevel,ComPaStopReason] = LevelLimitFunction1(OriginalPaVentLevel,VentAdj_PasCmdFaultSts, LocalPassengerHeatValid,VentAdj_CarType,VentAdj_HeatMsgLostFlag,VentAdj_RecoverDefaultFlag);
    [Com3rdVentLevel,Com3rdStopReason] = LevelLimitFunction2(Original3rdVentLevel,VentAdj_ThirdCmdFaultSts, LocalThirdHeatValid,VentAdj_CarType,VentAdj_HeatMsgLostFlag,VentAdj_RecoverDefaultFlag);
    settings: executionOrder=2
  state [Level,StopReason] = LevelLimitFunction1(OriginalLevel,Error,OppositeCmd,CarType,Vent_CanMessageLostFlag,Vent_RecoverDefaultFlag) [function]
  state [Level,StopReason] = LevelLimitFunction2(OriginalLevel,Error,OppositeCmd,CarType,Vent_CanMessageLostFlag,Vent_RecoverDefaultFlag) [function]
  state [Level,TimeoutFlag] = TimeoutFunction(TimeoutPrm,MaxTime,InLevel) [function]
  state TimeLimitDeal [parallel]
    en,du:
    [TimeDrVentLevel,TimeoutDrFlag] = TimeoutFunction(VentAdj_TimeOutPrm,VentRunMaxTime,ComDrVentLevel);
    [TimePaVentLevel,TimeoutPaFlag] = TimeoutFunction1(VentAdj_TimeOutPrm,VentRunMaxTime,ComPaVentLevel);
    [Time3rdVentLevel,Timeout3rdFlag] = TimeoutFunction2(VentAdj_TimeOutPrm,VentRunMaxTime,Com3rdVentLevel);
    settings: executionOrder=3
  state [Level,TimeoutFlag] = TimeoutFunction1(TimeoutPrm,MaxTime,InLevel) [function]
  state [Level,TimeoutFlag] = TimeoutFunction2(TimeoutPrm,MaxTime,InLevel) [function]
  state StopReason = StopFunction(ComStop,Timeout) [function]
  state StopReasonDeal [parallel]
    en,du:
    [DrVentStopReason] = StopFunction(ComDrStopReason,TimeoutDrFlag);
    [PaVentStopReason] = StopFunction1(ComPaStopReason,TimeoutPaFlag);
    [ThirdHeatStopReason] = StopFunction2(Com3rdStopReason,Timeout3rdFlag);
    settings: executionOrder=4
  state StopReason = StopFunction1(ComStop,Timeout) [function]
  state StopReason = StopFunction2(ComStop,Timeout) [function]
  state [Level,Type] = DiagnoseFunction(DiagCommand,InLevel,CurrentType) [function]
  state DiagnoseCtrlDeal [parallel]
    en,du:
    [DiagDrVentLevel,VentDriverRunType] = DiagnoseFunction(VentAdj_DriverDiagCmd,TimeDrVentLevel,OrgVentDriverRunType);
    [DiagPaVentLevel,VentPassengerRunType] = DiagnoseFunction1(VentAdj_PassengerDiagCmd,TimePaVentLevel, OrgVentPassengerRunType);
    [Diag3rdVentLevel,VentThirdRunType] = DiagnoseFunction2(VentAdj_ThirdDiagCmd,Time3rdVentLevel,OrgVentThirdRunType);
    settings: executionOrder=5
  state [Level,Type] = DiagnoseFunction1(DiagCommand,InLevel,CurrentType) [function]
  state [Level,Type] = DiagnoseFunction2(DiagCommand,InLevel,CurrentType) [function]
  data: MixFlg function_input uint8; Valid function_input uint8; OutValid function_output; OriginalLevel function_input; Error function_input; OppositeCmd function_input; CarType function_input; Level function_output; StopReason function_output; Vent_CanMessageLostFlag function_input; Vent_RecoverDefaultFlag function_input; OriginalLevel function_input; Error function_input; OppositeCmd function_input; CarType function_input; Level function_output; StopReason function_output; Vent_CanMessageLostFlag function_input; Vent_RecoverDefaultFlag function_input; OriginalLevel function_input; Error function_input; OppositeCmd function_input; CarType function_input; Level function_output; StopReason function_output; Vent_CanMessageLostFlag function_input; Vent_RecoverDefaultFlag function_input; TimeoutPrm function_input; MaxTime function_input uint32; InLevel function_input; Level function_output; TimeoutFlag function_output; TimeoutPrm function_input; MaxTime function_input uint32; InLevel function_input; Level function_output; TimeoutFlag function_output; TimeoutPrm function_input; MaxTime function_input uint32; InLevel function_input; Level function_output; TimeoutFlag function_output; ComStop function_input; Timeout function_input; StopReason function_output; ComStop function_input; Timeout function_input; StopReason function_output; ComStop function_input; Timeout function_input; StopReason function_output; DiagCommand function_input; InLevel function_input; Level function_output; CurrentType function_input; Type function_output; DiagCommand function_input; InLevel function_input; Level function_output; CurrentType function_input; Type function_output; DiagCommand function_input; InLevel function_input; Level function_output; CurrentType function_input; Type function_output; OriginalDrVentLevel input; OriginalPaVentLevel input; Original3rdVentLevel input; VentAdj_VoltMode input; VentAdj_DriverCmdFaultSts input; VentAdj_PasCmdFaultSts input; VentAdj_ThirdCmdFaultSts input; DriverHeatValid input; PassengerHeatValid input; ThirdHeatValid input; VentAdj_CarType input; VentAdj_RecoverDefaultFlag input; VentAdj_HeatMsgLostFlag input; VentAdj_TimeOutPrm input; VentRunMaxTime input; ComDrVentLevel local Enum: enVentLvlSts; ComPaVentLevel local Enum: enVentLvlSts; Com3rdVentLevel local Enum: enVentLvlSts; TimeDrVentLevel local Enum: enVentLvlSts; TimePaVentLevel local Enum: enVentLvlSts; Time3rdVentLevel local Enum: enVentLvlSts; ComDrStopReason local Enum: enVentStopReason; ComPaStopReason local Enum: enVentStopReason; Com3rdStopReason local Enum: enVentStopReason; TimeoutDrFlag local uint8; TimeoutPaFlag local uint8; Timeout3rdFlag local uint8; DrVentStopReason output Enum: enVentStopReason; ThirdHeatStopReason output Enum: enVentStopReason; PaVentStopReason output Enum: enVentStopReason; DiagDrVentLevel output Enum: enVentLvlSts; DiagPaVentLevel output Enum: enVentLvlSts; Diag3rdVentLevel output Enum: enVentLvlSts; VentDriverRunType output Enum: enVentType; VentPassengerRunType output Enum: enVentType; VentThirdRunType output Enum: enVentType; OrgVentDriverRunType input; OrgVentPassengerRunType input; OrgVentThirdRunType input; VentAdj_DriverDiagCmd input; VentAdj_PassengerDiagCmd input; VentAdj_ThirdDiagCmd input; Driver_MixConflicFlg input; Passenger_MixConflicFlg input; Third_MixConflicFlg input; LocalDriverHeatValid local uint8; LocalPassengerHeatValid local uint8; LocalThirdHeatValid local uint8

== stateflow chart Appl_VentAdj_CtrlModel/LogicCtrl/LocalAdjustCtrl/VentLevelDeal ==
  state [RunType,OutLevel] = VentRunTypeFunction(InLevel,PreLevel,InType) [function]
  state Level = LevelAquireFunction(EnableCfg,CarTypeCfg,PowerMode,EngineSts,CAN_Message,DisableSts,CAN_Lvl,Type) [function]
  state Level = LevelAquireFunction3(EnableCfg,CarTypeCfg,PowerMode,EngineSts,CAN_Message,DisableSts,CAN_Lvl,Type) [function]
  state Level = LevelAquireFunction1(EnableCfg,CarTypeCfg,PowerMode,EngineSts,CAN_Message,DisableSts,CAN_Lvl,Type) [function]
  state Level = LevelAquireFunction4(EnableCfg,CarTypeCfg,PowerMode,EngineSts,CAN_Message,DisableSts,CAN_Lvl,Type) [function]
  state Level = LevelAquireFunction2(EnableCfg,CarTypeCfg,PowerMode,EngineSts,CAN_Message,DisableSts,CAN_Lvl,Type) [function]
  state Level = LevelAquireFunction5(EnableCfg,CarTypeCfg,PowerMode,EngineSts,CAN_Message,DisableSts,CAN_Lvl,Type) [function]
  state DriverVentLevelDeal [parallel]
    settings: executionOrder=1
    state Tbox_VentFunction [parallel]
      settings: executionOrder=2
      (default) -> (junction 65)
      DriverVentLevelDeal.Tbox_VentFunction -> (junction 65)
      (junction 65) -> (junction 67) [order 1] : [TRUE == RemoteModeFlag]
      (junction 65) -> (junction 355) [order 2]
      (junction 67) -> (junction 62) : {LocalDrTboxVentLevel = LevelAquireFunction3(VentAdj_DriverEnableConfig, ...
          | VentAdj_CarType,VentAdj_PowerMode,ComPCSatisfiedFlag, ...
          | DriverTbox_VentMessage,VentAdj_DrVentStopReason,VentAdj_CanDrvVentLvl,TRUE);}
      (junction 355) -> (junction 176)
      (junction 62) -> (junction 359) : {[OrgVentDriverRunType,OriginalDrVentLevel] = VentRunTypeFunction ...
          | (LocalDrTboxVentLevel,OriginalDrVentLevel,enVentType.EN_VENT_TYPE_TBOX);}
      (junction 359) -> (junction 176)
      (junction 176) -> (junction 70)
    state HMI_VentFunction [parallel]
      settings: executionOrder=1
      (default) -> (junction 163)
      DriverVentLevelDeal.HMI_VentFunction -> (junction 163)
      (junction 163) -> (junction 39) : {LocalVentDrHMILevel = LevelAquireFunction(VentAdj_DriverEnableConfig, ...
          | VentAdj_CarType,VentAdj_PowerMode,ComPCSatisfiedFlag, ...
          | DriverHMI_VentMessage,VentAdj_DrVentStopReason,VentAdj_CanDrvVentLvl,FALSE);}
      (junction 39) -> (junction 45) : {[OrgVentDriverRunType,OriginalDrVentLevel] = VentRunTypeFunction ...
          | (LocalVentDrHMILevel,OriginalDrVentLevel,enVentType.EN_VENT_TYPE_HMI);}
      (junction 45) -> (junction 329)
  state PassengerVentLevelDeal [parallel]
    settings: executionOrder=2
    state HMI_VentFunction [parallel]
      settings: executionOrder=1
      (default) -> (junction 222)
      PassengerVentLevelDeal.HMI_VentFunction -> (junction 222)
      (junction 222) -> (junction 221) : {LocalVentPaHMILevel = LevelAquireFunction1(VentAdj_PassengerEnableConfig, ...
          | VentAdj_CarType,VentAdj_PowerMode,ComPCSatisfiedFlag, ...
          | PassengerHMI_VentMessage,VentAdj_PaVentStopReason,VentAdj_CanPasVentLvl,FALSE);}
      (junction 221) -> (junction 218) : {[OrgVentPassengerRunType,OriginalPaVentLevel] = VentRunTypeFunction ...
          | (LocalVentPaHMILevel,OriginalPaVentLevel,enVentType.EN_VENT_TYPE_HMI);}
      (junction 218) -> (junction 213)
    state Tbox_VentFunction [parallel]
      settings: executionOrder=2
      (default) -> (junction 209)
      PassengerVentLevelDeal.Tbox_VentFunction -> (junction 209)
      (junction 209) -> (junction 250) [order 1] : [TRUE == RemoteModeFlag]
      (junction 209) -> (junction 246) [order 2]
      (junction 250) -> (junction 206) : {LocalPaTboxVentLevel = LevelAquireFunction4(VentAdj_PassengerEnableConfig, ...
          | VentAdj_CarType,VentAdj_PowerMode,ComPCSatisfiedFlag, ...
          | PassengerTbox_VentMessage,VentAdj_PaVentStopReason,VentAdj_CanPasVentLvl,TRUE);}
      (junction 206) -> (junction 194) : {[OrgVentPassengerRunType,OriginalPaVentLevel] = VentRunTypeFunction ...
          | (LocalPaTboxVentLevel,OriginalPaVentLevel,enVentType.EN_VENT_TYPE_TBOX);}
      (junction 194) -> (junction 246)
      (junction 246) -> (junction 231)
  state ThirdVentLevelDeal [parallel]
    settings: executionOrder=3
    state HMI_VentFunction [parallel]
      settings: executionOrder=1
      (default) -> (junction 254)
      ThirdVentLevelDeal.HMI_VentFunction -> (junction 254)
      (junction 254) -> (junction 265) : {LocalVent3rdHMILevel = LevelAquireFunction2(VentAdj_ThirdEnableConfig, ...
          | VentAdj_CarType,VentAdj_PowerMode,ComPCSatisfiedFlag, ...
          | ThirdHMI_VentMessage,VentAdj_ThirdVentStopReason,VentAdj_CanThirdVentLvl,FALSE);}
      (junction 265) -> (junction 255) : {[OrgVentThirdRunType,Original3rdVentLevel] = VentRunTypeFunction ...
          | (LocalVent3rdHMILevel,Original3rdVentLevel,enVentType.EN_VENT_TYPE_HMI);}
      (junction 255) -> (junction 261)
    state Tbox_VentFunction [parallel]
      settings: executionOrder=2
      (default) -> (junction 270)
      ThirdVentLevelDeal.Tbox_VentFunction -> (junction 270)
      (junction 270) -> (junction 293) [order 1] : [TRUE == RemoteModeFlag]
      (junction 270) -> (junction 295) [order 2]
      (junction 293) -> (junction 275) : {LocalVent3rdTboxLevel = LevelAquireFunction5(VentAdj_ThirdEnableConfig, ...
          | VentAdj_CarType,VentAdj_PowerMode,ComPCSatisfiedFlag, ...
          | ThirdTbox_VentMessage,VentAdj_ThirdVentStopReason,VentAdj_CanThirdVentLvl,TRUE);}
      (junction 275) -> (junction 304) : {[OrgVentThirdRunType,Original3rdVentLevel] = VentRunTypeFunction ...
          | (LocalVent3rdTboxLevel,Original3rdVentLevel,enVentType.EN_VENT_TYPE_TBOX);}
      (junction 304) -> (junction 295)
      (junction 295) -> (junction 258)
  data: InLevel function_input; RunType function_output; PreLevel function_input; InType function_input; OutLevel function_output; EnableCfg function_input; Level function_output; CarTypeCfg function_input; PowerMode function_input; EngineSts function_input; CAN_Message function_input; DisableSts function_input; CAN_Lvl function_input; Type function_input uint8; EnableCfg function_input; Level function_output; CarTypeCfg function_input; PowerMode function_input; EngineSts function_input; CAN_Message function_input; DisableSts function_input; CAN_Lvl function_input; Type function_input uint8; EnableCfg function_input; Level function_output; CarTypeCfg function_input; PowerMode function_input; EngineSts function_input; CAN_Message function_input; DisableSts function_input; CAN_Lvl function_input; Type function_input uint8; EnableCfg function_input; Level function_output; CarTypeCfg function_input; PowerMode function_input; EngineSts function_input; CAN_Message function_input; DisableSts function_input; CAN_Lvl function_input; Type function_input uint8; EnableCfg function_input; Level function_output; CarTypeCfg function_input; PowerMode function_input; EngineSts function_input; CAN_Message function_input; DisableSts function_input; CAN_Lvl function_input; Type function_input uint8; EnableCfg function_input; Level function_output; CarTypeCfg function_input; PowerMode function_input; EngineSts function_input; CAN_Message function_input; DisableSts function_input; CAN_Lvl function_input; Type function_input uint8; VentAdj_DriverEnableConfig input; VentAdj_PassengerEnableConfig input; VentAdj_ThirdEnableConfig input; VentAdj_DrVentStopReason input; VentAdj_PaVentStopReason input; VentAdj_ThirdVentStopReason input; VentAdj_PowerMode input; VentAdj_CarType input; DriverHMI_VentMessage input; DriverTbox_VentMessage input; PassengerHMI_VentMessage input; PassengerTbox_VentMessage input; ThirdHMI_VentMessage input; ThirdTbox_VentMessage input; OriginalDrVentLevel output Enum: enVentLvlSts; OrgVentDriverRunType output Enum: enVentType; ComPCSatisfiedFlag input; RemoteModeFlag input; TRUE parameter; OriginalPaVentLevel output Enum: enVentLvlSts; OrgVentPassengerRunType output Enum: enVentType; Original3rdVentLevel output Enum: enVentLvlSts; OrgVentThirdRunType output Enum: enVentType; LocalDrTboxVentLevel local uint8 =255; LocalPaTboxVentLevel local uint8 =255; LocalVent3rdTboxLevel local uint8 =255; LocalVentDrHMILevel local uint8 =255; LocalVentPaHMILevel local uint8 =255; LocalVent3rdHMILevel local uint8 =255; VentAdj_CanDrvVentLvl input; VentAdj_CanPasVentLvl input; VentAdj_CanThirdVentLvl input; FALSE parameter

== stateflow chart Appl_VentAdj_CtrlModel/LogicCtrl/LocalAdjustCtrl/LimitDeal/LevelLimitFunction1/LevelLimit ==
  state Default
    en:
    Level = enVentLvlSts.EN_VENT_LVL_OFF;
  state Run
    en:
    Level = OriginalLevel;
    du:
    Level = OriginalLevel;
  state ForbidStatus
    en:
    Level = enVentLvlSts.EN_VENT_LVL_OFF;
    ex:
    StopReason = enVentStopReason.EN_VENT_STOP_R_NONE;
    (default) -> (junction 74)
    ForbidStatus -> (junction 74) [order 1]
    (junction 74) -> (junction 46) [order 1] : /*存在故障*/
        | [enVentCmdFault.EN_VENT_FAULT_NONE != Error]
    (junction 74) -> (junction 71) [order 2]
    (junction 46) -> (junction 60) : {StopReason = enVentStopReason.EN_VENT_STOP_R_FAULT;}
    (junction 60) -> (junction 71)
    (junction 71) -> (junction 70)
    (junction 70) -> (junction 43) [order 1] : /*互斥命令有效*/
        | [TRUE == OppositeCmd]
    (junction 70) -> (junction 54) [order 2]
    (junction 43) -> (junction 49) : {StopReason = enVentStopReason.EN_VENT_STOP_R_CMD;}
    (junction 49) -> (junction 54)
    (junction 54) -> (junction 59)
    (junction 59) -> (junction 78) [order 1] : /*恢复出厂*/
        | [TRUE == Vent_RecoverDefaultFlag]
    (junction 59) -> (junction 57) [order 2]
    (junction 78) -> (junction 42) : {StopReason = enVentStopReason.EN_VENT_STOP_R_FACTORY;}
    (junction 42) -> (junction 57)
    (junction 57) -> (junction 51)
    (junction 51) -> (junction 48) [order 1] : /*BM400掉线禁能*/
        | [TRUE == Vent_CanMessageLostFlag && enProjectType.EN_PROJECT_BM400 == CarType]
    (junction 51) -> (junction 40) [order 2]
    (junction 48) -> (junction 65) : {StopReason = enVentStopReason.EN_VENT_STOP_R_LOSS;}
    (junction 65) -> (junction 40)
    (junction 40) -> (junction 68)
  (default) -> Default
  ForbidStatus -> Default [order 1] : /*无用户请求，可准备下一轮禁能原因检测*/
      | [enVentLvlSts.EN_VENT_LVL_OFF == OriginalLevel]
  Default -> ForbidStatus : /*请求工作*/
      | [enVentLvlSts.EN_VENT_LVL_OFF != OriginalLevel]
  Run -> ForbidStatus [commented out] : /*非正常电压模式*/
      | [enFinalPowerMode.EN_NORMAL_VOLT != VoltMode]
      | /StopReason = enVentStopReason.EN_VENT_STOP_R_VOL;
  Run -> ForbidStatus [order 1] : /*存在故障*/
      | [enVentCmdFault.EN_VENT_FAULT_NONE != Error]
      | /StopReason = enVentStopReason.EN_VENT_STOP_R_FAULT;
  Run -> ForbidStatus [order 2] : /*互斥命令有效*/
      | [TRUE == OppositeCmd]
      | /StopReason = enVentStopReason.EN_VENT_STOP_R_CMD;
  Run -> ForbidStatus [order 3] : /*恢复出厂*/
      | [TRUE == Vent_RecoverDefaultFlag]
      | /StopReason = enVentStopReason.EN_VENT_STOP_R_FACTORY;
  Run -> ForbidStatus [order 4] : /*BM400掉线禁能*/
      | [TRUE == Vent_CanMessageLostFlag && enProjectType.EN_PROJECT_BM400 == CarType]
      | /StopReason = enVentStopReason.EN_VENT_STOP_R_LOSS;
  ForbidStatus -> Run [order 2] : /*无故障
      | && 互斥命令无效
      | && 无恢复出厂命令
      | && （BM400控制报文在线 || 非BM400车型）*/
      | [enVentCmdFault.EN_VENT_FAULT_NONE == Error ...
      | && TRUE != OppositeCmd ...
      | && TRUE != Vent_RecoverDefaultFlag ...
      | && ((FALSE == Vent_CanMessageLostFlag && enProjectType.EN_PROJECT_BM400 == CarType) ...
      | || (enProjectType.EN_PROJECT_BM400 != CarType))]
  data: Level output Enum: enVentLvlSts; StopReason output Enum: enVentStopReason; OriginalLevel input Enum: enVentLvlSts; Error input uint8; CarType input Enum: enProjectType; TRUE parameter; OppositeCmd input uint8; Vent_CanMessageLostFlag input uint8; Vent_RecoverDefaultFlag input uint8; FALSE parameter
